simulink model "danche2758s"  (R2021a)
settings: Solver=VariableStepAuto  StartTime=0.0  StopTime=20  RelTol=1e-3
model workspace (MAT data in the model file):
  v_follow = 1
libraries: simulink x9, rllib x1
settings Model: Creator=ROBOT  LastModifiedBy=hp
settings SolverCC: AlgebraicLoopSolver=TrustRegion
settings DebuggingCC: UnconnectedInputMsg=none  UnconnectedOutputMsg=none  UnconnectedLineMsg=none  ArithmeticOperatorsInVariantConditions=warning
settings ModelReferenceCC: EnableRefExpFcnMdlSchedulingChecks=off
settings SFSimCC: CustomCodeUndefinedFunction=UseInterfaceOnly
settings RTWCC: Description=Generic Real-Time Target  DLArmComputeVersion=20.02.1

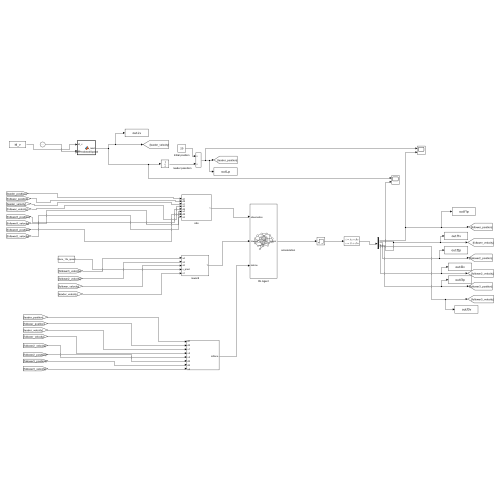
[thumbnail: Simulink's stored preview of the top-level diagram]
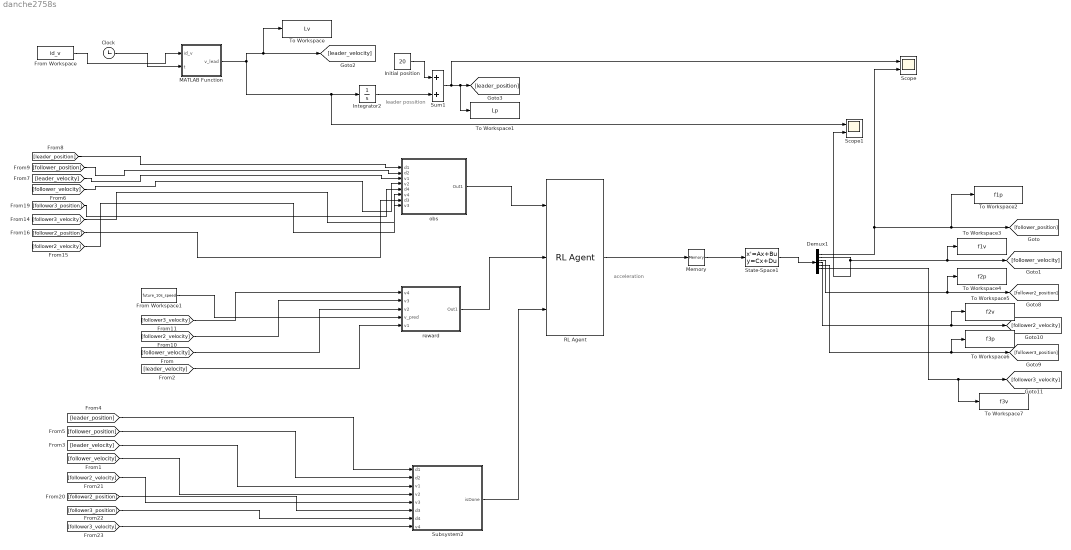
== system danche2758s ==
  note: leader possition
  note: acceleration
  Clock : Clock
  Demux1 : Demux  Outputs=6
  From Workspace : FromWorkspace  VariableName=id_v  OutDataTypeStr=double  OutputAfterFinalValue=Holding final value
  From Workspace1 : FromWorkspace  VariableName=future_10s_speed  OutDataTypeStr=double  ZeroCross=off  OutputAfterFinalValue=Holding final value
  Initial position : Constant  Value=20
  Integrator2 : Integrator
  MATLAB Function : MATLAB Function  TreatAsAtomicUnit=on
  Memory : Memory  InitialCondition=[0,0,0]'
  RL Agent : rllib/RL Agent  Agent=agent  ExternalActionAsInput=off  ProvideLastAction=off  ProvideCumRwd=off  TreatAsDirectFeedthrough=on  UseStrictObservationDataTypes=off
  Scope : Scope  NumInputPorts=2
  Scope1 : Scope  NumInputPorts=2
  State-Space1 : StateSpace  A=[0 1 0 0 0 0; 0 0 0 0 0 0; 0 0 0 1 0 0; 0 0 0 0 0 0; 0 0 0 0 0 1; 0 0 0 0 0 0]  B=[0 0 0 ; 1 0 0 ; 0 0 0 ; 0 1 0 ; 0 0 0 ; 0 0 1 ]  C=[1 0 0 0 0 0; 0 1 0 0 0 0; 0 0 1 0 0 0; 0 0 0 1 0 0; 0 0 0 0 1 0; 0 0 0 0 0 1]  D=[0 0 0; 0 0 0; 0 0 0; 0 0 0; 0 0 0; 0 0 0]  InitialCondition=[ 10, 40, 0, 40, -10, 40 ]'  ParameterTunability=Unconstrained
  Subsystem2 : Subsystem
  Sum1 : Sum
  To Workspace : ToWorkspace  VariableName=Lv  SampleTime=-1
      settings: Save2DSignal=2-D array (concatenate along first dimension)
  To Workspace1 : ToWorkspace  VariableName=Lp  SampleTime=-1
      settings: Save2DSignal=2-D array (concatenate along first dimension)
  To Workspace2 : ToWorkspace  VariableName=f1p  SampleTime=-1
      settings: Save2DSignal=2-D array (concatenate along first dimension)
  To Workspace3 : ToWorkspace  VariableName=f1v  SampleTime=-1
      settings: Save2DSignal=2-D array (concatenate along first dimension)
  To Workspace4 : ToWorkspace  VariableName=f2p  SampleTime=-1
      settings: Save2DSignal=2-D array (concatenate along first dimension)
  To Workspace5 : ToWorkspace  VariableName=f2v  SampleTime=-1
      settings: Save2DSignal=2-D array (concatenate along first dimension)
  To Workspace6 : ToWorkspace  VariableName=f3p  SampleTime=-1
      settings: Save2DSignal=2-D array (concatenate along first dimension)
  To Workspace7 : ToWorkspace  VariableName=f3v  SampleTime=-1
      settings: Save2DSignal=2-D array (concatenate along first dimension)
  obs : Subsystem
  reward : Subsystem
  wires:
  Memory/1 -> State-Space1/1
  State-Space1/1 -> Demux1/1
  Demux1/1 -> To Workspace2/1, [follower_position], Scope/2
  Demux1/2 -> To Workspace3/1, [follower_velocity], Scope1/2
  [follower_velocity] -> Subsystem2/4(v2)
  Initial position/1 -> Sum1/1
  Integrator2/1 -> Sum1/2
  Sum1/1 -> Scope/1, To Workspace1/1, [leader_position]
  [leader_velocity] -> Subsystem2/3(v1)
  [leader_position] -> Subsystem2/1(d1)
  [follower_position] -> Subsystem2/2(d2)
  reward/1(Out1) -> RL Agent/2
  [leader_velocity] -> reward/5(v1)
  [follower_velocity] -> reward/3(v2)
  [follower2_velocity] -> reward/2(v3)
  [follower3_velocity] -> reward/1(v4)
  obs/1(Out1) -> RL Agent/1
  [leader_position] -> obs/1(d1)
  [follower_position] -> obs/2(d2)
  [leader_velocity] -> obs/3(v1)
  [follower_velocity] -> obs/4(v2)
  [follower2_velocity] -> obs/8(v3)
  [follower3_velocity] -> obs/6(v4)
  [follower2_position] -> obs/7(d3)
  [follower3_position] -> obs/5(d4)
  Subsystem2/1(isDone) -> RL Agent/3
  [follower2_position] -> Subsystem2/6(d3)
  [follower2_velocity] -> Subsystem2/5(v3)
  [follower3_position] -> Subsystem2/7(d4)
  [follower3_velocity] -> Subsystem2/8(v4)
  Demux1/3 -> To Workspace4/1, [follower2_position]
  Demux1/4 -> To Workspace5/1, [follower2_velocity]
  Demux1/5 -> To Workspace6/1, [follower3_position]
  Demux1/6 -> To Workspace7/1, [follower3_velocity]
  RL Agent/1 -> Memory/1
  MATLAB Function/1(v_lead) -> To Workspace/1, [leader_velocity], Scope1/1, Integrator2/1
  Clock/1 -> MATLAB Function/2(t)
  From Workspace/1 -> MATLAB Function/1(id_v)
  From Workspace1/1 -> reward/4(v_pred)

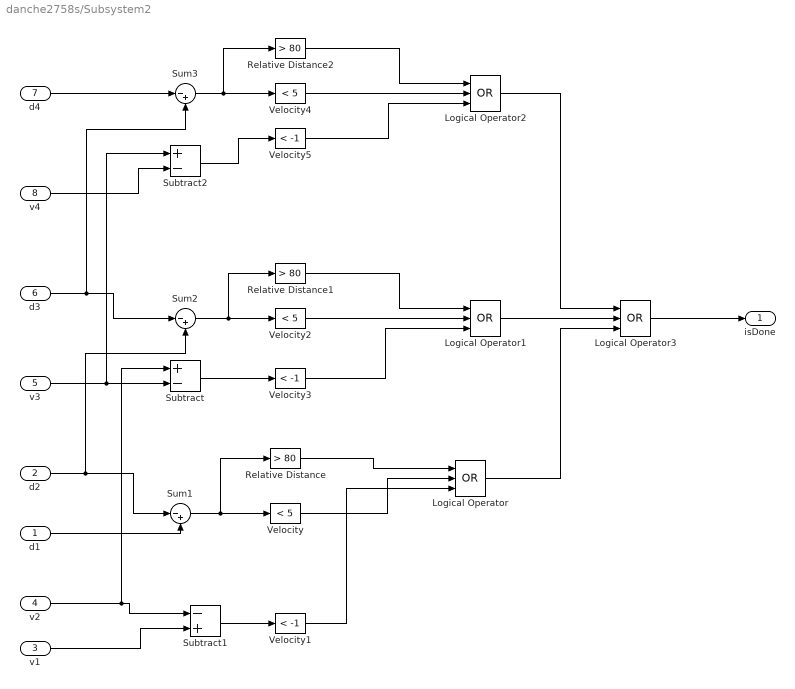
== system danche2758s/Subsystem2 ==
  d1 : Inport
  d2 : Inport  Port=2
  v1 : Inport  Port=3
  v2 : Inport  Port=4
  v3 : Inport  Port=5
  d3 : Inport  Port=6
  d4 : Inport  Port=7
  v4 : Inport  Port=8
  Logical Operator{,1..3} (4 alike) : Logic  Operator=OR  Inputs=3  AllPortsSameDT=off  OutDataTypeStr=boolean
  Relative Distance : simulink/Logic and Bit Operations/Compare To Constant  relop=>  const=80  OutDataTypeStr=boolean
  Relative Distance1 : simulink/Logic and Bit Operations/Compare To Constant  relop=>  const=80  OutDataTypeStr=boolean
  Relative Distance2 : simulink/Logic and Bit Operations/Compare To Constant  relop=>  const=80  OutDataTypeStr=boolean
  Subtract : Sum  Inputs=+-
  Subtract1 : Sum  Inputs=-+
  Subtract2 : Sum  Inputs=+-
  Sum1 : Sum  Inputs=|-+  SaturateOnIntegerOverflow=on
  Sum2 : Sum  Inputs=|-+  SaturateOnIntegerOverflow=on
  Sum3 : Sum  Inputs=|-+  SaturateOnIntegerOverflow=on
  Velocity : simulink/Logic and Bit Operations/Compare To Constant  relop=<  const=5  OutDataTypeStr=boolean
  Velocity1 : simulink/Logic and Bit Operations/Compare To Constant  relop=<  const=-1  OutDataTypeStr=boolean
  Velocity2 : simulink/Logic and Bit Operations/Compare To Constant  relop=<  const=5  OutDataTypeStr=boolean
  Velocity3 : simulink/Logic and Bit Operations/Compare To Constant  relop=<  const=-1  OutDataTypeStr=boolean
  Velocity4 : simulink/Logic and Bit Operations/Compare To Constant  relop=<  const=5  OutDataTypeStr=boolean
  Velocity5 : simulink/Logic and Bit Operations/Compare To Constant  relop=<  const=-1  OutDataTypeStr=boolean
  isDone : Outport
  wires:
  Velocity1/1 -> Logical Operator/3
  v2/1 -> Subtract1/1, Subtract/1
  Sum1/1 -> Velocity/1, Relative Distance/1
  Relative Distance/1 -> Logical Operator/1
  Velocity/1 -> Logical Operator/2
  d1/1 -> Sum1/2
  d2/1 -> Sum1/1, Sum2/2
  v3/1 -> Subtract2/1, Subtract/2
  Subtract/1 -> Velocity3/1
  v1/1 -> Subtract1/2
  Subtract1/1 -> Velocity1/1
  Velocity3/1 -> Logical Operator1/3
  d3/1 -> Sum2/1, Sum3/2
  Sum2/1 -> Relative Distance1/1, Velocity2/1
  Relative Distance1/1 -> Logical Operator1/1
  Velocity2/1 -> Logical Operator1/2
  Relative Distance2/1 -> Logical Operator2/1
  Velocity4/1 -> Logical Operator2/2
  Velocity5/1 -> Logical Operator2/3
  Sum3/1 -> Relative Distance2/1, Velocity4/1
  Subtract2/1 -> Velocity5/1
  d4/1 -> Sum3/1
  v4/1 -> Subtract2/2
  Logical Operator2/1 -> Logical Operator3/1
  Logical Operator1/1 -> Logical Operator3/2
  Logical Operator/1 -> Logical Operator3/3
  Logical Operator3/1 -> isDone/1

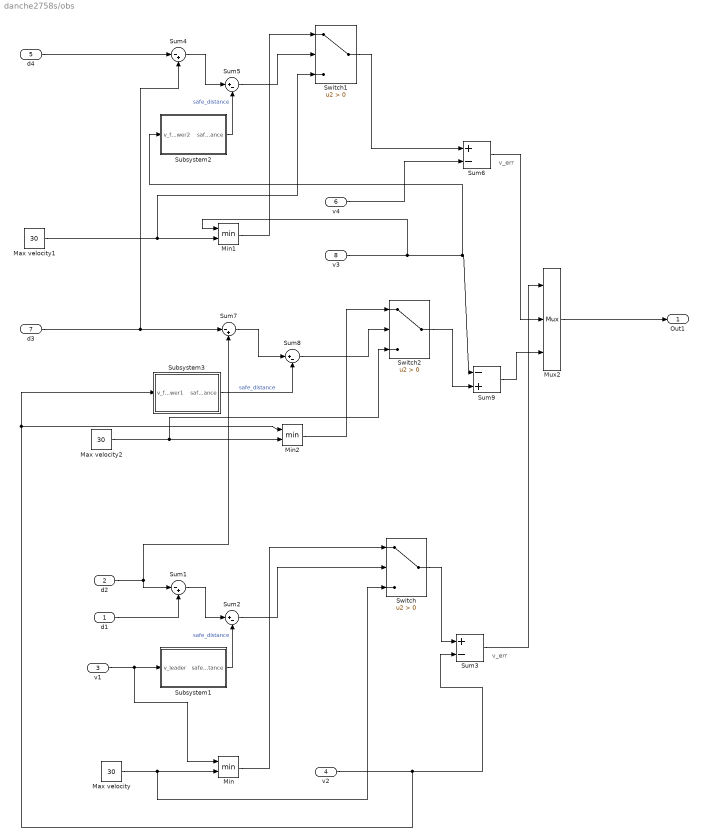
== system danche2758s/obs ==
  note: v_err
  note: v_err
  d1 : Inport
  d2 : Inport  Port=2
  v1 : Inport  Port=3
  v2 : Inport  Port=4
  d4 : Inport  Port=5
  v4 : Inport  Port=6
  d3 : Inport  Port=7
  v3 : Inport  Port=8
  Max velocity : Constant  Value=30
  Max velocity1 : Constant  Value=30
  Max velocity2 : Constant  Value=30
  Min : MinMax  Inputs=2
  Min1 : MinMax  Inputs=2
  Min2 : MinMax  Inputs=2
  Mux2 : Mux  Inputs=3
  Subsystem1 : Subsystem
  Subsystem2 : Subsystem
  Subsystem3 : Subsystem
  Sum1 : Sum  Inputs=|-+  SaturateOnIntegerOverflow=on
  Sum2 : Sum  Inputs=|+-  SaturateOnIntegerOverflow=on
  Sum3 : Sum  Inputs=+-
  Sum4 : Sum  Inputs=|-+  SaturateOnIntegerOverflow=on
  Sum5 : Sum  Inputs=|+-  SaturateOnIntegerOverflow=on
  Sum6 : Sum  Inputs=+-
  Sum7 : Sum  Inputs=|-+  SaturateOnIntegerOverflow=on
  Sum8 : Sum  Inputs=|+-  SaturateOnIntegerOverflow=on
  Sum9 : Sum  Inputs=-+
  Switch : Switch  Criteria=u2 > Threshold
  Switch1 : Switch  Criteria=u2 > Threshold
  Switch2 : Switch  Criteria=u2 > Threshold
  Out1 : Outport
  wires:
  v1/1 -> Min/1, Subsystem1/1(v_leader)
  d2/1 -> Sum7/2, Sum1/1
  d1/1 -> Sum1/2
  Sum1/1 -> Sum2/1
  Subsystem1/1(safe_distance) -> Sum2/2  "safe_distance"
  Sum2/1 -> Switch/2
  Min/1 -> Switch/1
  Max velocity/1 -> Switch/3, Min/2
  Switch/1 -> Sum3/1
  v2/1 -> Sum3/2, Min2/1, Subsystem3/1(v_follower1)
  d4/1 -> Sum4/1
  Min1/1 -> Switch1/1
  Max velocity1/1 -> Switch1/3, Min1/2
  Subsystem2/1(safe_distance) -> Sum5/2  "safe_distance"
  Sum5/1 -> Switch1/2
  Sum4/1 -> Sum5/1
  Switch1/1 -> Sum6/1
  v4/1 -> Sum6/2
  d3/1 -> Sum4/2, Sum7/1
  Sum7/1 -> Sum8/1
  Subsystem3/1(safe_distance) -> Sum8/2  "safe_distance"
  Max velocity2/1 -> Switch2/3, Min2/2
  Min2/1 -> Switch2/1
  Sum8/1 -> Switch2/2
  Switch2/1 -> Sum9/2
  Mux2/1 -> Out1/1
  Sum9/1 -> Mux2/3
  v3/1 -> Min1/1, Subsystem2/1(v_follower2), Sum9/1
  Sum6/1 -> Mux2/2
  Sum3/1 -> Mux2/1

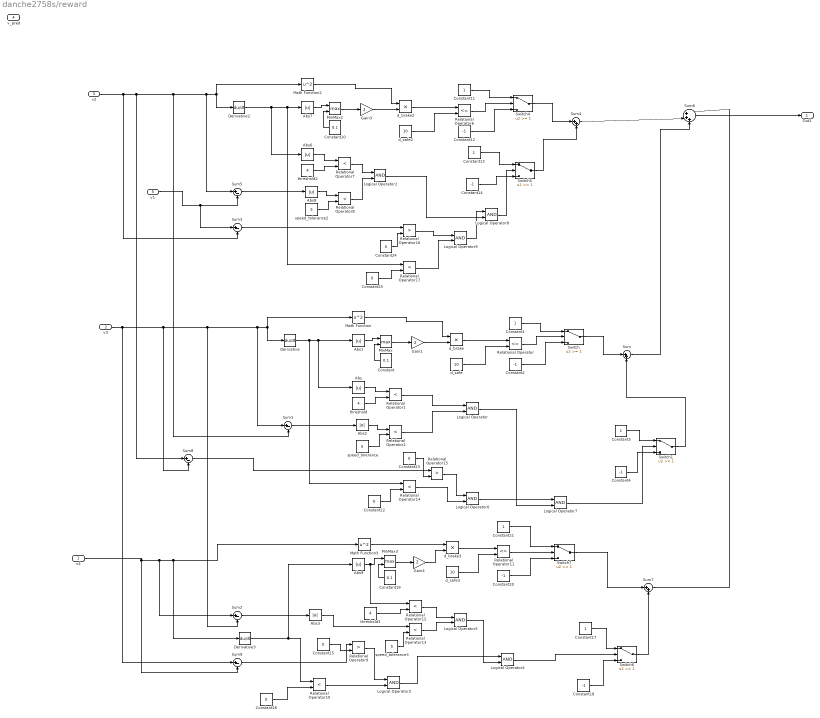
== system danche2758s/reward ==
  v4 : Inport
  v3 : Inport  Port=2
  v2 : Inport  Port=3
  v_pred : Inport  Port=4
  v1 : Inport  Port=5
  Abs{,1..3,6..9} (8 alike) : Abs  ZeroCross=off
  Constant : Constant  Value=0.1
  Constant{1,3,11,13,17,21} (6 alike) : Constant
  Constant10 : Constant  Value=0.1
  Constant{2,4,12,14,18,20} (6 alike) : Constant  Value=-1
  Constant{15..16,22..25} (6 alike) : Constant  Value=0
  Constant19 : Constant  Value=0.1
  Derivative : Derivative
  Derivative2 : Derivative
  Derivative3 : Derivative
  Gain1 : Gain  Gain=2
  Gain3 : Gain  Gain=2
  Gain4 : Gain  Gain=2
  Logical Operator{,2..9} (9 alike) : Logic  AllPortsSameDT=off  OutDataTypeStr=boolean
  Math Function : Math  Operator=square  SaturateOnIntegerOverflow=on
  Math Function2 : Math  Operator=square  SaturateOnIntegerOverflow=on
  Math Function3 : Math  Operator=square  SaturateOnIntegerOverflow=on
  MinMax : MinMax  Function=max  Inputs=2  ZeroCross=off
  MinMax2 : MinMax  Function=max  Inputs=2  ZeroCross=off
  MinMax3 : MinMax  Function=max  Inputs=2  ZeroCross=off
  Relational Operator : RelationalOperator  Operator=<=  OutDataTypeStr=boolean  ZeroCross=off  RndMeth=Simplest
  Relational Operator{1..2,7..8,10,12..14,17} (9 alike) : RelationalOperator  Operator=<  OutDataTypeStr=boolean  ZeroCross=off  RndMeth=Simplest
  Relational Operator11 : RelationalOperator  Operator=<=  OutDataTypeStr=boolean  ZeroCross=off  RndMeth=Simplest
  Relational Operator15 : RelationalOperator  Operator=>  OutDataTypeStr=boolean  ZeroCross=off  RndMeth=Simplest
  Relational Operator16 : RelationalOperator  Operator=>  OutDataTypeStr=boolean  ZeroCross=off  RndMeth=Simplest
  Relational Operator6 : RelationalOperator  Operator=<=  OutDataTypeStr=boolean  ZeroCross=off  RndMeth=Simplest
  Relational Operator9 : RelationalOperator  Operator=>  OutDataTypeStr=boolean  ZeroCross=off  RndMeth=Simplest
  Sum : Sum  Inputs=|++
  Sum{1..3,5,8..9} (6 alike) : Sum  Inputs=|+-
  Sum4 : Sum  Inputs=|++
  Sum6 : Sum  Inputs=|+++
  Sum7 : Sum  Inputs=|++
  Switch{,1,4..7} (6 alike) : Switch  Threshold=1  ZeroCross=off
  d_brake : Product
  d_brake2 : Product
  d_brake3 : Product
  d_safe : Constant  Value=10
  d_safe2 : Constant  Value=10
  d_safe3 : Constant  Value=10
  speed_tolerance : Constant  Value=5
  speed_tolerance2 : Constant  Value=5
  speed_tolerance3 : Constant  Value=5
  threshold : Constant  Value=4
  threshold2 : Constant  Value=4
  threshold3 : Constant  Value=4
  Out1 : Outport
  wires:
  Abs1/1 -> MinMax/1
  Constant/1 -> MinMax/2
  Math Function/1 -> d_brake/1
  MinMax/1 -> Gain1/1
  Gain1/1 -> d_brake/2
  d_brake/1 -> Relational Operator/1
  d_safe/1 -> Relational Operator/2
  Relational Operator/1 -> Switch/2
  Constant1/1 -> Switch/1
  Constant2/1 -> Switch/3
  Abs/1 -> Relational Operator1/1
  threshold/1 -> Relational Operator1/2
  Abs2/1 -> Relational Operator2/1
  speed_tolerance/1 -> Relational Operator2/2
  Relational Operator1/1 -> Logical Operator/1
  Relational Operator2/1 -> Logical Operator/2
  Constant3/1 -> Switch1/1
  Constant4/1 -> Switch1/3
  Switch/1 -> Sum/1
  Derivative/1 -> Relational Operator14/1, Abs/1, Abs1/1
  Sum1/1 -> Abs2/1
  Gain3/1 -> d_brake2/2
  MinMax2/1 -> Gain3/1
  Math Function2/1 -> d_brake2/1
  Abs7/1 -> MinMax2/1
  Relational Operator7/1 -> Logical Operator2/1
  speed_tolerance2/1 -> Relational Operator8/2
  threshold2/1 -> Relational Operator7/2
  d_brake2/1 -> Relational Operator6/1
  Relational Operator6/1 -> Switch4/2
  Constant10/1 -> MinMax2/2
  Relational Operator8/1 -> Logical Operator2/2
  Constant14/1 -> Switch5/3
  Abs6/1 -> Relational Operator7/1
  Constant13/1 -> Switch5/1
  d_safe2/1 -> Relational Operator6/2
  Switch5/1 -> Sum4/2
  Switch4/1 -> Sum4/1
  Derivative2/1 -> Abs6/1, Relational Operator17/1, Abs7/1
  Constant11/1 -> Switch4/1
  Abs8/1 -> Relational Operator8/1
  Constant12/1 -> Switch4/3
  Sum5/1 -> Abs8/1
  Sum/1 -> Sum6/3
  Sum4/1 -> Sum6/2
  Sum6/1 -> Out1/1
  Constant15/1 -> Relational Operator9/2
  Constant16/1 -> Relational Operator10/2
  Derivative3/1 -> Abs9/1, Relational Operator10/1
  Relational Operator9/1 -> Logical Operator3/1
  Relational Operator10/1 -> Logical Operator3/2
  Constant17/1 -> Switch6/1
  Constant18/1 -> Switch6/3
  Math Function3/1 -> d_brake3/1
  Abs9/1 -> Relational Operator12/1, MinMax3/1
  Constant19/1 -> MinMax3/2
  MinMax3/1 -> Gain4/1
  Gain4/1 -> d_brake3/2
  d_brake3/1 -> Relational Operator11/1
  d_safe3/1 -> Relational Operator11/2
  Relational Operator11/1 -> Switch7/2
  Constant20/1 -> Switch7/3
  Constant21/1 -> Switch7/1
  Switch7/1 -> Sum7/1
  Switch6/1 -> Sum7/2
  Logical Operator3/1 -> Logical Operator4/1
  threshold3/1 -> Relational Operator12/2
  Relational Operator12/1 -> Logical Operator5/1
  Relational Operator13/1 -> Logical Operator5/2
  Logical Operator5/1 -> Logical Operator4/2
  Logical Operator4/1 -> Switch6/2
  speed_tolerance3/1 -> Relational Operator13/2
  Constant22/1 -> Relational Operator14/2
  Relational Operator14/1 -> Logical Operator6/2
  Relational Operator15/1 -> Logical Operator6/1
  Constant23/1 -> Relational Operator15/2
  Logical Operator6/1 -> Logical Operator7/1
  Logical Operator/1 -> Logical Operator7/2
  Logical Operator7/1 -> Switch1/2
  Switch1/1 -> Sum/2
  Logical Operator8/1 -> Switch5/2
  Logical Operator2/1 -> Logical Operator8/2
  Logical Operator9/1 -> Logical Operator8/1
  Relational Operator16/1 -> Logical Operator9/1
  Constant24/1 -> Relational Operator16/2
  Relational Operator17/1 -> Logical Operator9/2
  Constant25/1 -> Relational Operator17/2
  v1/1 -> Sum3/1, Sum5/2
  Sum2/1 -> Abs3/1
  Abs3/1 -> Relational Operator13/1
  v2/1 -> Sum3/2, Sum8/1, Sum1/2, Derivative2/1, Math Function2/1, Sum5/1
  Sum3/1 -> Relational Operator16/1
  Sum8/1 -> Relational Operator15/1
  v4/1 -> Sum9/2, Sum2/1, Derivative3/1, Math Function3/1
  v3/1 -> Sum9/1, Sum8/2, Sum2/2, Sum1/1, Derivative/1, Math Function/1
  Sum9/1 -> Relational Operator9/1
  Sum7/1 -> Sum6/1

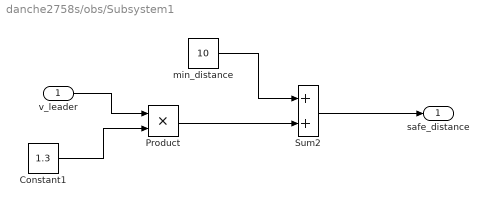
== system danche2758s/obs/Subsystem1 ==
  v_leader : Inport
  Constant1 : Constant  Value=1.3
  Product : Product
  Sum2 : Sum
  "min_distance " : Constant  Value=10
  safe_distance : Outport  VectorParamsAs1DForOutWhenUnconnected=off
  wires:
  v_leader/1 -> Product/1
  "min_distance "/1 -> Sum2/1
  Constant1/1 -> Product/2
  Product/1 -> Sum2/2
  Sum2/1 -> safe_distance/1

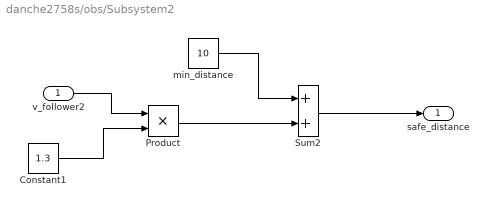
== system danche2758s/obs/Subsystem2 ==
  v_follower2 : Inport
  Constant1 : Constant  Value=1.3
  Product : Product
  Sum2 : Sum
  "min_distance " : Constant  Value=10
  safe_distance : Outport  VectorParamsAs1DForOutWhenUnconnected=off
  wires:
  v_follower2/1 -> Product/1
  "min_distance "/1 -> Sum2/1
  Constant1/1 -> Product/2
  Product/1 -> Sum2/2
  Sum2/1 -> safe_distance/1

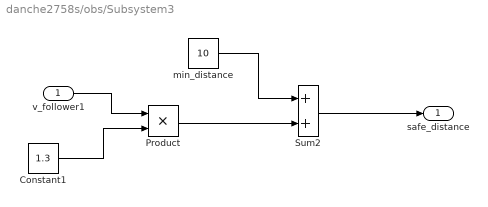
== system danche2758s/obs/Subsystem3 ==
  v_follower1 : Inport
  Constant1 : Constant  Value=1.3
  Product : Product
  Sum2 : Sum
  "min_distance " : Constant  Value=10
  safe_distance : Outport  VectorParamsAs1DForOutWhenUnconnected=off
  wires:
  v_follower1/1 -> Product/1
  "min_distance "/1 -> Sum2/1
  Constant1/1 -> Product/2
  Product/1 -> Sum2/2
  Sum2/1 -> safe_distance/1

== matlab function danche2758s/MATLAB Function ==
  data: id_v input; t input; v_lead output
function v_lead = getPredictedSpeed(id_v, t)
%#codegen

% 计算索引，假设 t 从 1 开始，每秒对应一行数据
index = round(t)+1;

% 确保索引在有效范围内
if index > 0 && index <= size(id_v, 1)
    v_lead = id_v(index);  % 直接获取对应秒数的速度值
else
    v_lead = id_v(end); % 如果索引超出范围，返回最后一个有效预测值
end
end
